simulink model "lineal_model_discreto"  (R2015a)
settings: Solver=ode45  StartTime=0.0  StopTime=2  RelTol=1e-3
values from neighbouring files (symbols this model uses):
  A = A1    [Final_2.m]    (also in Final_discreto.m)
  Aod = Aaumd-Ld*Caumd    [Final_discreto.m]
  B = B1    [Final_2.m]    (also in Final_discreto.m)
  Bod = [Baumd Ld]    [Final_discreto.m]
  Cod = [eye(size(Aod,1)-1) zeros(size(Aod,1)-1,1)]    [Final_discreto.m]
  Dod = zeros(size(Aod,1)-1,2)    [Final_discreto.m]
  kid = kd(5,1)    [Final_discreto.m]
  ksd = [kd(1,1) kd(2,1) kd(3,1) kd(4,1) ]'    [Final_discreto.m]
  Ts = 1/(50e3)    (= 2e-05)    [Final_2.m]    (also in Final_discreto.m)
settings Model: Creator=berme_000  LastModifiedBy=berme_000

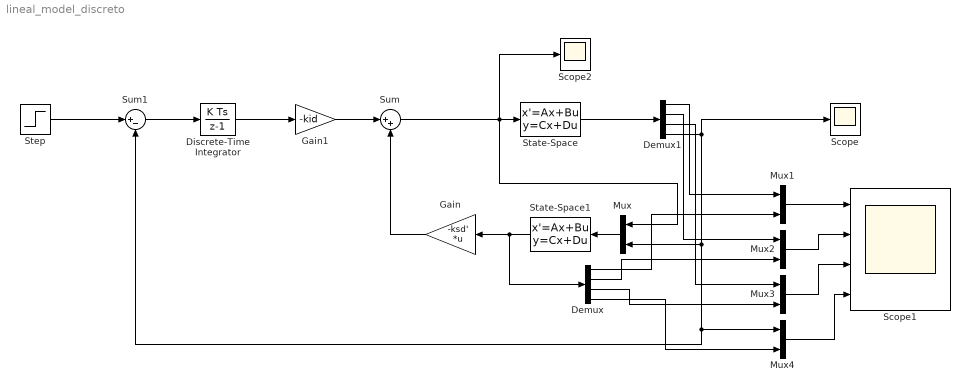
== system lineal_model_discreto ==
  Demux : Demux
  Demux1 : Demux
  Discrete-Time Integrator : DiscreteIntegrator  InitialConditionSetting=State (most efficient)  SampleTime=Ts
  Gain : Gain  Gain=-ksd'  Multiplication=Matrix(K*u)
  Gain1 : Gain  Gain=-kid
  Mux{,1..4} (5 alike) : Mux  Inputs=2
  Scope : Scope
      settings: TimeRange=2  YMin=-45000000000000  YMax=5000000000000
  Scope1 : Scope  NumInputPorts=4
      settings: YMin=-8.13152e-20~-0.00075~-5~-5  YMax=0.0015~0.00075~5~5
  Scope2 : Scope
      settings: YMin=-0.5  YMax=10  SaveName=ScopeData2
  State-Space : StateSpace  A=A  B=B  C=eye(4)  D=zeros(4,1)  X0=[.1 -.1 .2 -.1]
  State-Space1 : StateSpace  A=Aod  B=Bod  C=Cod  D=Dod  X0=0
  Step : Step  Time=0.5  After=5  SampleTime=0
  Sum : Sum  Inputs=|++
  Sum1 : Sum  Inputs=|+-
  wires:
  Demux1/4 -> Scope/1, Mux/2, Mux4/1, Sum1/2
  Mux/1 -> State-Space1/1
  State-Space1/1 -> Demux/1, Gain/1
  Discrete-Time Integrator/1 -> Gain1/1
  Gain1/1 -> Sum/1
  Gain/1 -> Sum/2
  Sum1/1 -> Discrete-Time Integrator/1
  Step/1 -> Sum1/1
  Mux1/1 -> Scope1/1
  Mux2/1 -> Scope1/2
  Mux3/1 -> Scope1/3
  Mux4/1 -> Scope1/4
  Demux1/1 -> Mux1/1
  Demux/1 -> Mux1/2
  Demux1/2 -> Mux2/1
  Demux1/3 -> Mux3/1
  Demux/2 -> Mux2/2
  Demux/3 -> Mux3/2
  Demux/4 -> Mux4/2
  Sum/1 -> Mux/1, Scope2/1, State-Space/1
  State-Space/1 -> Demux1/1
